simulink model "t5"  (R2016a)
settings: Solver=VariableStepAuto  StartTime=0.0  StopTime=10.0  RelTol=1e-3
settings Model: Creator=admin  LastModifiedBy=admin

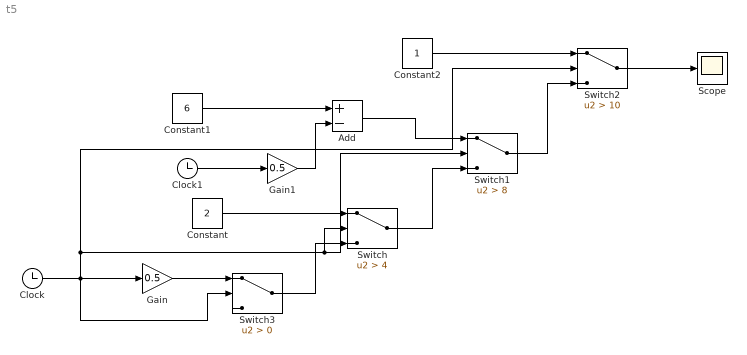
== system t5 ==
  Add : Sum  Inputs=+-
  Clock : Clock
  Clock1 : Clock
  Constant : Constant  Value=2
  Constant1 : Constant  Value=6
  Constant2 : Constant
  Gain : Gain  Gain=0.5
  Gain1 : Gain  Gain=0.5
  Scope : Scope
  Switch : Switch  Criteria=u2 > Threshold  Threshold=4
  Switch1 : Switch  Criteria=u2 > Threshold  Threshold=8
  Switch2 : Switch  Criteria=u2 > Threshold  Threshold=10
  Switch3 : Switch  Criteria=u2 > Threshold
  wires:
  Clock/1 -> Switch2/2, Switch1/2, Switch/2, Switch3/2, Gain/1
  Gain/1 -> Switch3/1
  Switch3/1 -> Switch/3
  Switch/1 -> Switch1/3
  Switch1/1 -> Switch2/3
  Constant/1 -> Switch/1
  Clock1/1 -> Gain1/1
  Gain1/1 -> Add/2
  Constant1/1 -> Add/1
  Add/1 -> Switch1/1
  Constant2/1 -> Switch2/1
  Switch2/1 -> Scope/1
